simulink subsystem "Time_Flag"  (R2022b)
settings: Solver=VariableStepAuto  StartTime=0.0  StopTime=10.0  RelTol=1e-3
settings Model: Creator=User  LastModifiedBy=User

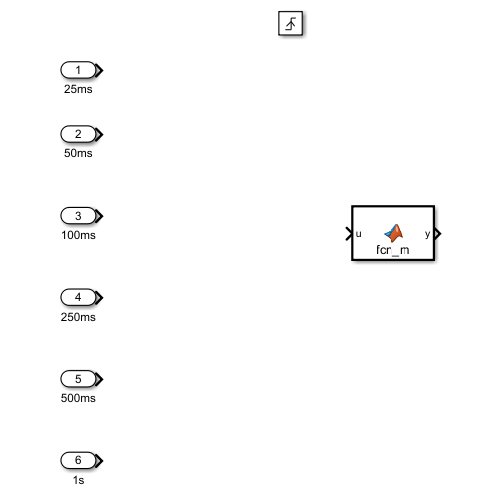
[thumbnail: Simulink's stored preview of the top-level diagram]
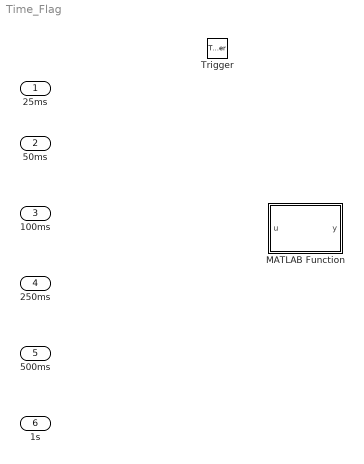
== system Time_Flag ==
  25ms : Inport
  50ms : Inport  Port=2
  100ms : Inport  Port=3
  250ms : Inport  Port=4
  500ms : Inport  Port=5
  1s : Inport  Port=6
  Trigger : TriggerPort  VariantControl=(inherit)  PortDimensions=1
  MATLAB Function : MATLAB Function  TreatAsAtomicUnit=on

== matlab function Time_Flag/MATLAB Function ==
  data: u input; y output
function y = fcn_m(u)
    y = fcn(u);
    
end
